simulink model "remoteMicrogrid"  (R2023a)
settings: Solver=FixedStepDiscrete  StartTime=0.0  StopTime=8  FixedStep=Ts  RelTol=1e-3
PreLoadFcn:
  | remoteMicrogridInputData
undefined symbols (not defined in the file): BESS, ControlRoom, DiscIntNeverNeededParam, Grid, Load, Machine, Microgrid, PV, T_on, Ts
libraries: ee_lib x46, eeGeneralControl x35, nesl_utility_internal x25, simulink x24, nesl_utility x20, fl_lib x17, slpidlib x12, eeTransforms x5, eeRmsMeasurement x4, eeTotalHarmonicDistorsion x4, eeSinusoidalMeasurement x3, batteryecm_lib x2
(part 5 of 5)

== system remoteMicrogrid/Operator Control Room/Measurements and visualizations /Resynchronization and Planned Islanding/Planned Islanding ==
  Grid Frequency : Inport
  Island Frequency : Inport  Port=2
  Grid Current : Inport  Port=3
  Island Voltage : Inport  Port=4
  Grid Voltage1 : Inport  Port=5
  PlannedIslandCommand : Inport  Port=6
  PlannedIsland : Inport  Port=7
  Power Tracking Command : Inport  Port=8
  BRK : Inport  Port=9
  " Grid and Island Voltage Frequency " : Scope  NumInputPorts=2
  Bus Creator1 : BusCreator  Inputs=2
  Bus Creator2 : BusCreator  Inputs=2
  Bus Creator3 : BusCreator  Inputs=4
  Bus Creator4 : BusCreator  Inputs=2
  "Grid Active & Reactive Power " : Subsystem
  Grid Voltage2 : InportShadow  Port=5
  Planned Islanding PCC voltage,Current : Scope  NumInputPorts=4
  wires:
  Bus Creator4/1 -> Planned Islanding PCC voltage,Current/4
  Bus Creator3/1 -> Planned Islanding PCC voltage,Current/1
  PlannedIslandCommand/1 -> Bus Creator3/1
  Grid Voltage2/1 -> Planned Islanding PCC voltage,Current/3, "Grid Active & Reactive Power "/1(Vabc)  "Grid Voltage"
  "Grid Active & Reactive Power "/2(Q) -> Bus Creator4/2  "Reactive Power (pu)"
  Grid Current/1 -> Planned Islanding PCC voltage,Current/2, "Grid Active & Reactive Power "/2(Iabc)
  "Grid Active & Reactive Power "/1(P) -> Bus Creator4/1  "Active Power (pu)"
  PlannedIsland/1 -> Bus Creator3/2
  Grid Frequency/1 -> Bus Creator1/1  "Grid Frequency"
  Island Frequency/1 -> Bus Creator1/2  "Island Frequency"
  Bus Creator1/1 -> " Grid and Island Voltage Frequency "/1
  Bus Creator2/1 -> " Grid and Island Voltage Frequency "/2
  Grid Voltage1/1 -> Bus Creator2/1  "Grid Voltage"
  Island Voltage/1 -> Bus Creator2/2  "Island Voltage"
  Power Tracking Command/1 -> Bus Creator3/3
  BRK/1 -> Bus Creator3/4

== system remoteMicrogrid/Operator Control Room/Measurements and visualizations /Resynchronization and Planned Islanding/Resync ==
  Grid Frequency : Inport
  Island Frequency : Inport  Port=2
  In1 : Inport  Port=3
  Grid Angle : Inport  Port=4
  Island Angle : Inport  Port=5
  Resynchronization : Inport  Port=6
  Grid Voltage : Inport  Port=7
  Grid Current : Inport  Port=8
  Island Voltage : Inport  Port=9
  Frequency Error : Inport  Port=10
  Grid Voltage1 : Inport  Port=11
  Phase Angle Error : Inport  Port=12
  Voltage Error : Inport  Port=13
  Bus Creator{,1..4} (5 alike) : BusCreator  Inputs=2
  "Grid Active & Reactive Power " : Subsystem
  Resynch and PCC voltage,Current : Scope  NumInputPorts=4
  Voltage and Frequency Matching : Scope  NumInputPorts=6
  wires:
  Grid Current/1 -> Resynch and PCC voltage,Current/2, "Grid Active & Reactive Power "/2(Iabc)
  Bus Creator1/1 -> Voltage and Frequency Matching/2
  Resynchronization/1 -> Bus Creator3/2
  Bus Creator3/1 -> Resynch and PCC voltage,Current/1
  "Grid Active & Reactive Power "/1(P) -> Bus Creator4/1  "Active Power (pu)"
  Island Voltage/1 -> Bus Creator2/2
  Grid Voltage1/1 -> Resynch and PCC voltage,Current/3, "Grid Active & Reactive Power "/1(Vabc)
  Bus Creator4/1 -> Resynch and PCC voltage,Current/4
  Bus Creator2/1 -> Voltage and Frequency Matching/3
  Bus Creator/1 -> Voltage and Frequency Matching/1
  Grid Frequency/1 -> Bus Creator/1
  Grid Angle/1 -> Bus Creator1/1
  Voltage Error/1 -> Voltage and Frequency Matching/6
  Island Frequency/1 -> Bus Creator/2
  Island Angle/1 -> Bus Creator1/2
  Phase Angle Error/1 -> Voltage and Frequency Matching/5
  Grid Voltage/1 -> Bus Creator2/1
  "Grid Active & Reactive Power "/2(Q) -> Bus Creator4/2  "Reactive Power (pu)"
  In1/1 -> Bus Creator3/1  "Resynch Command"
  Frequency Error/1 -> Voltage and Frequency Matching/4

== system remoteMicrogrid/Operator Control Room/Monitoring of system performance/Load /Subsystem4 ==
  Voltage : Inport
  Change Detector : eeGeneralControl/Change Detector  VariantControl=Variant1  LabelModeActiveChoice=Discrete  ChangeType=Rising edge  x0=0  Ts=Ts
  Change Detector1 : eeGeneralControl/Change Detector  VariantControl=Variant1  LabelModeActiveChoice=Discrete  ChangeType=Rising edge  x0=0  Ts=Ts
  Compare To Constant2 : simulink/Logic and Bit Operations/Compare To Constant  relop=<=  const=Microgrid.LoadVolatgeRMSLow  OutDataTypeStr=boolean
  Compare To Constant3 : simulink/Logic and Bit Operations/Compare To Constant  relop=>  const=Microgrid.LoadVolatgeRMSHigh  OutDataTypeStr=boolean
  VoltageLow : Outport
  VoltageHigh : Outport  Port=2
  wires:
  Change Detector/1 -> VoltageLow/1
  Compare To Constant2/1 -> Change Detector/1
  Voltage/1 -> Compare To Constant3/1, Compare To Constant2/1
  Change Detector1/1 -> VoltageHigh/1
  Compare To Constant3/1 -> Change Detector1/1

== system remoteMicrogrid/Operator Control Room/Monitoring of system performance/Load /start at 0.2 s2 ==
  In1 : Inport
  Constant : Constant  Value=0.707
  Step : Step  Time=0.3  SampleTime=Ts
  Switch : Switch  Criteria=u2 > Threshold  Threshold=0.5  SaturateOnIntegerOverflow=off  InputSameDT=off
  u : Outport
  wires:
  In1/1 -> Switch/1
  Switch/1 -> u/1
  Constant/1 -> Switch/3
  Step/1 -> Switch/2

== system remoteMicrogrid/Operator Control Room/Monitoring of system performance/Load /start at 0.2 s4 ==
  In1 : Inport
  Constant : Constant  Value=0.491
  Step : Step  Time=0.3  SampleTime=Ts
  Switch : Switch  Criteria=u2 > Threshold  Threshold=0.5  SaturateOnIntegerOverflow=off  InputSameDT=off
  u : Outport
  wires:
  In1/1 -> Switch/1
  Switch/1 -> u/1
  Constant/1 -> Switch/3
  Step/1 -> Switch/2

== system remoteMicrogrid/Operator Control Room/Monitoring of system performance/Load /start at 0.2 s5 ==
  In1 : Inport
  Constant : Constant  Value=75
  Step : Step  Time=0.3  SampleTime=Ts
  Switch : Switch  Criteria=u2 > Threshold  Threshold=0.5  SaturateOnIntegerOverflow=off  InputSameDT=off
  u : Outport
  wires:
  Step/1 -> Switch/2
  Constant/1 -> Switch/3
  Switch/1 -> u/1
  In1/1 -> Switch/1

== system remoteMicrogrid/Operator Control Room/Monitoring of system performance/Microgrid/Subsystem ==
  Frequency : Inport
  Change Detector : eeGeneralControl/Change Detector  VariantControl=Variant1  LabelModeActiveChoice=Discrete  ChangeType=Rising edge  x0=0  Ts=Ts
  Change Detector1 : eeGeneralControl/Change Detector  VariantControl=Variant1  LabelModeActiveChoice=Discrete  ChangeType=Rising edge  x0=0  Ts=Ts
  Compare To Constant2 : simulink/Logic and Bit Operations/Compare To Constant  relop=<  const=Microgrid.FrequencyLow  OutDataTypeStr=boolean
  Compare To Constant3 : simulink/Logic and Bit Operations/Compare To Constant  relop=>  const=Microgrid.FrequencyHigh  OutDataTypeStr=boolean
  FrequencyLow : Outport
  FrequencyHigh : Outport  Port=2
  wires:
  Change Detector/1 -> FrequencyLow/1
  Compare To Constant2/1 -> Change Detector/1
  Frequency/1 -> Compare To Constant3/1, Compare To Constant2/1
  Change Detector1/1 -> FrequencyHigh/1
  Compare To Constant3/1 -> Change Detector1/1

== system remoteMicrogrid/Operator Control Room/Monitoring of system performance/Microgrid/Subsystem3 ==
  Voltage : Inport
  Change Detector : eeGeneralControl/Change Detector  VariantControl=Variant1  LabelModeActiveChoice=Discrete  ChangeType=Rising edge  x0=0  Ts=Ts
  Change Detector1 : eeGeneralControl/Change Detector  VariantControl=Variant1  LabelModeActiveChoice=Discrete  ChangeType=Rising edge  x0=0  Ts=Ts
  Compare To Constant2 : simulink/Logic and Bit Operations/Compare To Constant  relop=<=  const=Microgrid.VoltageLow  OutDataTypeStr=boolean
  Compare To Constant3 : simulink/Logic and Bit Operations/Compare To Constant  relop=>  const=Microgrid.VoltageHigh  OutDataTypeStr=boolean
  VoltageLow : Outport
  VoltageHigh : Outport  Port=2
  wires:
  Compare To Constant3/1 -> Change Detector/1
  Change Detector/1 -> VoltageHigh/1
  Voltage/1 -> Compare To Constant2/1, Compare To Constant3/1
  Compare To Constant2/1 -> Change Detector1/1
  Change Detector1/1 -> VoltageLow/1

== system remoteMicrogrid/Operator Control Room/Monitoring of system performance/Microgrid/start at 2 s ==
  In1 : Inport
  Constant : Constant  Value=60
  Step : Step  Time=2  SampleTime=Ts
  Switch : Switch  Criteria=u2 > Threshold  Threshold=0.5  SaturateOnIntegerOverflow=off  InputSameDT=off
  u : Outport
  wires:
  Step/1 -> Switch/2
  Constant/1 -> Switch/3
  Switch/1 -> u/1
  In1/1 -> Switch/1

== system remoteMicrogrid/Operator Control Room/Monitoring of system performance/Microgrid/start at 2 s1 ==
  In1 : Inport
  Constant : Constant
  Step : Step  Time=2  SampleTime=Ts
  Switch : Switch  Criteria=u2 > Threshold  Threshold=0.5  SaturateOnIntegerOverflow=off  InputSameDT=off
  u : Outport
  wires:
  Step/1 -> Switch/2
  Constant/1 -> Switch/3
  Switch/1 -> u/1
  In1/1 -> Switch/1

== system remoteMicrogrid/Operator Control Room/Monitoring of system performance/Subsystem/start at 2.5 s ==
  ReactivePower : Inport
  Constant : Constant
  Step : Step  Time=2.5  SampleTime=Ts
  Switch : Switch  Criteria=u2 > Threshold  Threshold=0.5  SaturateOnIntegerOverflow=off  InputSameDT=off
  u : Outport
  wires:
  ReactivePower/1 -> Switch/1
  Switch/1 -> u/1
  Constant/1 -> Switch/3
  Step/1 -> Switch/2

== system remoteMicrogrid/Operator Control Room/Monitoring of system performance/Subsystem/start at 2.5 s1 ==
  ActivePower : Inport
  Constant : Constant
  Step : Step  Time=2.5  SampleTime=Ts
  Switch : Switch  Criteria=u2 > Threshold  Threshold=0.5  SaturateOnIntegerOverflow=off  InputSameDT=off
  u : Outport
  wires:
  Step/1 -> Switch/2
  Constant/1 -> Switch/3
  Switch/1 -> u/1
  ActivePower/1 -> Switch/1

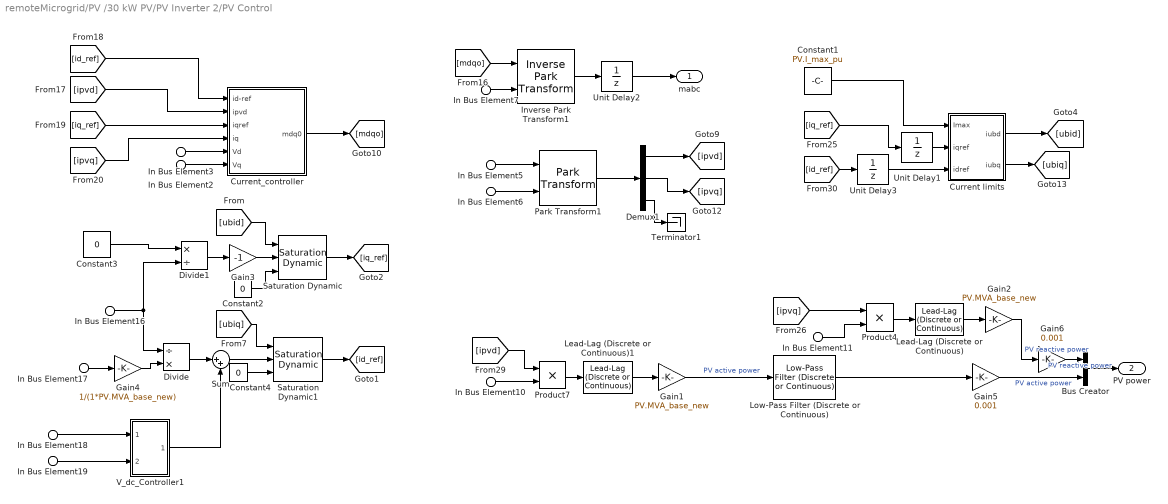
== system remoteMicrogrid/PV /30 kW PV/PV Inverter 2/PV Control ==
  In Bus Element17 : Inport  PortName=PV_plant1  Element=Pref1
  In Bus Element18 : Inport  PortName=PV_plant1  Element=Vdc_measured
  In Bus Element19 : Inport  PortName=PV_plant1  Element=Vdc_ref
  In Bus Element{3,10..11,16} (4 alike) : Inport  Port=2  PortName=PV  Element=Vd
  In Bus Element2 : Inport  Port=2  PortName=PV  Element=Vq
  In Bus Element6 : Inport  Port=2  PortName=PV  Element=Theta
  In Bus Element7 : Inport  Port=2  PortName=PV  Element=Theta
  In Bus Element5 : Inport  Port=3  PortName=ipv1  Element=1
  Bus Creator : BusCreator  Inputs=2
  Constant1 : Constant  Value=PV.I_max_pu
  Constant2 : Constant  Value=0
  Constant3 : Constant  Value=0
  Constant4 : Constant  Value=0
  Current limits : Subsystem
  Current_controller : Subsystem
  Demux1 : Demux  Outputs=3
  Divide : Product  Inputs=/*
  Divide1 : Product  Inputs=*/
  Gain1 : Gain  Gain=PV.MVA_base_new
  Gain2 : Gain  Gain=PV.MVA_base_new
  Gain3 : Gain  Gain=-1
  Gain4 : Gain  Gain=1/(1*PV.MVA_base_new)
  Gain5 : Gain  Gain=0.001
  Gain6 : Gain  Gain=0.001
  Inverse Park Transform1 : eeTransforms/Inverse Park Transform  AxisAlignment=Q-axis  PowerInvariant=off
  Lead-Lag (Discrete or Continuous) : eeGeneralControl/Lead-Lag (Discrete or Continuous)  T1=0  T2=PV.t_sensor  B=inf  A=-inf  init_option=Inherited from block input  x0=0  Ts=Ts
      settings: LibrarySourceBlock=|
      | ee_sl_lib/General Control/Lead-Lag
      | (Discrete or Continuous)
  Lead-Lag (Discrete or Continuous)1 : eeGeneralControl/Lead-Lag (Discrete or Continuous)  T1=0  T2=PV.t_sensor  B=inf  A=-inf  init_option=Inherited from block input  x0=0  Ts=Ts
      settings: LibrarySourceBlock=|
      | ee_sl_lib/General Control/Lead-Lag
      | (Discrete or Continuous)
  Low-Pass Filter (Discrete or Continuous) : eeGeneralControl/Low-Pass Filter (Discrete or Continuous)  K=1  T=0.02  B=inf  A=-inf  init_option=Inherited from block input  x0=0  Ts=-1
  Park Transform1 : eeTransforms/Park Transform  AxisAlignment=Q-axis  PowerInvariant=off
  Product4 : Product
  Product7 : Product
  Saturation Dynamic : simulink/Discontinuities/Saturation Dynamic  OutMin=[]  OutMax=[]  OutDataTypeStr=Inherit: Same as second input  OutDataType=fixdt(1, 16)  OutScaling=2^-10  DoSatur=off
  Saturation Dynamic1 : simulink/Discontinuities/Saturation Dynamic  OutMin=[]  OutMax=[]  OutDataTypeStr=Inherit: Same as second input  OutDataType=fixdt(1, 16)  OutScaling=2^-10  DoSatur=off
  Sum : Sum  Inputs=|++
  Terminator1 : Terminator
  Unit Delay1 : UnitDelay  SampleTime=Ts  HasFrameUpgradeWarning=on
  Unit Delay2 : UnitDelay  SampleTime=Ts  HasFrameUpgradeWarning=on
  Unit Delay3 : UnitDelay  SampleTime=Ts  HasFrameUpgradeWarning=on
  V_dc_Controller1 : Subsystem
  mabc : Outport
  PV power : Outport  Port=2
  wires:
  [id_ref] -> Unit Delay3/1
  Current limits/2(iubq) -> [ubiq]
  Gain1/1 -> Low-Pass Filter (Discrete or Continuous)/1  "PV active power"
  Product4/1 -> Lead-Lag (Discrete or Continuous)/1
  Product7/1 -> Lead-Lag (Discrete or Continuous)1/1
  In Bus Element2/1 -> Current_controller/6(Vq)
  Current_controller/1(mdq0) -> [mdqo]
  Constant1/1 -> Current limits/1(Imax)
  Inverse Park Transform1/1 -> Unit Delay2/1
  Demux1/2 -> [ipvq]
  Unit Delay2/1 -> mabc/1
  Demux1/1 -> [ipvd]
  [ipvq] -> Product4/1
  Demux1/3 -> Terminator1/1
  [mdqo] -> Inverse Park Transform1/1
  Current limits/1(iubd) -> [ubid]
  Park Transform1/1 -> Demux1/1
  [id_ref] -> Current_controller/1(id-ref)
  [iq_ref] -> Unit Delay1/1
  In Bus Element3/1 -> Current_controller/5(Vd)
  Unit Delay1/1 -> Current limits/2(iqref)
  [iq_ref] -> Current_controller/3(iqref)
  [ipvq] -> Current_controller/4(iq)
  In Bus Element10/1 -> Product7/2
  In Bus Element6/1 -> Park Transform1/2
  In Bus Element7/1 -> Inverse Park Transform1/2
  [ipvd] -> Product7/1
  Unit Delay3/1 -> Current limits/3(idref)
  In Bus Element11/1 -> Product4/2
  [ipvd] -> Current_controller/2(ipvd)
  Lead-Lag (Discrete or Continuous)1/1 -> Gain1/1
  Lead-Lag (Discrete or Continuous)/1 -> Gain2/1
  Gain2/1 -> Gain6/1  "PV reactive power"
  In Bus Element5/1 -> Park Transform1/1
  Constant4/1 -> Saturation Dynamic1/3
  V_dc_Controller1/1(Out1) -> Sum/2
  Constant2/1 -> Saturation Dynamic/3
  [ubiq] -> Saturation Dynamic1/1
  In Bus Element19/1 -> V_dc_Controller1/2(In2)
  Gain3/1 -> Saturation Dynamic/2
  In Bus Element18/1 -> V_dc_Controller1/1(PV_plant1)
  Gain4/1 -> Divide/2
  Sum/1 -> Saturation Dynamic1/2
  [ubid] -> Saturation Dynamic/1
  Constant3/1 -> Divide1/1
  In Bus Element16/1 -> Divide1/2, Divide/1
  Saturation Dynamic1/1 -> [id_ref]
  Divide/1 -> Sum/1
  Divide1/1 -> Gain3/1
  Saturation Dynamic/1 -> [iq_ref]
  In Bus Element17/1 -> Gain4/1
  Bus Creator/1 -> PV power/1
  Gain5/1 -> Bus Creator/2  "PV active power"
  Gain6/1 -> Bus Creator/1  "PV reactive power"
  Low-Pass Filter (Discrete or Continuous)/1 -> Gain5/1

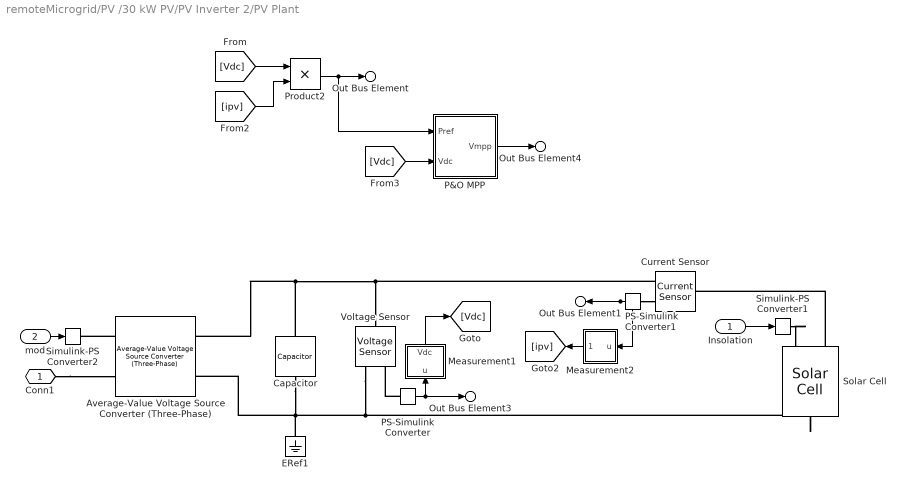
== system remoteMicrogrid/PV /30 kW PV/PV Inverter 2/PV Plant ==
  Insolation : Inport
  mod : Inport  Port=2
  Average-Value Voltage Source Converter (Three-Phase) : ee_lib/Semiconductors & Converters/Converters/Average-Value Voltage Source Converter (Three-Phase)  port_option=ee.enum.threePhasePort.composite  frequency_option=ee.enum.converters.frequency.variable  FRated=60 Hz  losses_parameterization=ee.enum.converters.losses.fixed  Pfixed=1 W  ks=0.01  kc1=1.7 V  kc2=0.01 Ohm  Ploss_vect=[100, 800, 1870, 3250, 4900] W  Irms_vect=[10, 100, 200, 300, 400] A  Vdc_nom=300 V  thermal_mass=30000 J/K  temperature_specify=off  temperature_priority=High  temperature=298.15 K  temperature_nominal_specify=off  temperature_nominal_unit=K  temperature_nominal_value=1
      settings: InternalSimscapePortConfiguration="{\"Bottom\":[],\"Left\":[{\"id\":\"ModWave\",\"label\":\"ModWave\",\"type\":\"input\"},{\"id\":\"N\",\"label\":\"~\",\"type\":\"foundation.electrical.three_phase\"}],\"Right\":[{\"id\":\"p\",\"label\":\"+\",\"type\":\"foundation.electrical.electrical\"},{\"id\":\"n\",\"label\":\"-\",\"type\":\"foundation.electrical.electrical\"}],\"Top\":[]}"
  Capacitor : fl_lib/Electrical/Electrical Elements/Capacitor  c=PV.C F  r=1e-6 Ohm  g=0 1/Ohm  i_specify=off  i_priority=None  i=0 A  i_nominal_specify=off  i_nominal_unit=A  i_nominal_value=1  v_specify=off  v_priority=None  v=6560*.5 V  v_nominal_specify=off  v_nominal_unit=V  v_nominal_value=1  vc_specify=on  vc_priority=None  vc=PV.Vdc V  vc_nominal_specify=off  vc_nominal_unit=V  vc_nominal_value=1
  Current Sensor : fl_lib/Electrical/Electrical Sensors/Current Sensor
  ERef1 : fl_lib/Electrical/Electrical Elements/Electrical Reference
  Measurement1 : Subsystem
  Measurement2 : Subsystem
  P&O MPP : Subsystem
  PS-Simulink Converter : nesl_utility/PS-Simulink Converter  PhysicalDomain=network_engine_domain  SubClassName=ps_output  LeftPortType=input  RightPortType=output  PseudoPeriodic=off  Frequencies=[]  VectorFormat=inherit  Unit=inherit  AffineConversion=off
  PS-Simulink Converter1 : nesl_utility/PS-Simulink Converter  PhysicalDomain=network_engine_domain  SubClassName=ps_output  LeftPortType=input  RightPortType=output  PseudoPeriodic=off  Frequencies=[]  VectorFormat=inherit  Unit=inherit  AffineConversion=off
  Product2 : Product
  Simulink-PS Converter1 : nesl_utility/Simulink-PS Converter  PhysicalDomain=network_engine_domain  SubClassName=ps_input  LeftPortType=input  RightPortType=output  PseudoPeriodic=off  Frequencies=[]  NoiseDistribution=none  NoiseParameters=[]  Unit=1  AffineConversion=off  FilteringAndDerivatives=provide  SimscapeFilterOrder=1  InputFilterTimeConstant=0.001  UdotUserProvided=0
  Simulink-PS Converter2 : nesl_utility/Simulink-PS Converter  PhysicalDomain=network_engine_domain  SubClassName=ps_input  LeftPortType=input  RightPortType=output  PseudoPeriodic=off  Frequencies=[]  NoiseDistribution=none  NoiseParameters=[]  Unit=1  AffineConversion=off  FilteringAndDerivatives=provide  SimscapeFilterOrder=1  InputFilterTimeConstant=0.001  UdotUserProvided=0
  Solar Cell : ee_lib/Sources/Solar Cell  prm=3  Isc=3.8 A  Voc=0.586 V  Is=Solar_cell.diode_saturation_current A  Is2=0 A  Iph=Solar_cell.solar_generated_current_AM A  Ir0=1000 W/m^2  ec=Solar_cell.quality_factor_i  N2=Solar_cell.quality_factor_j  Rs=Solar_cell.series_resistance Ohm  Rp=Solar_cell.parallel_resistance Ohm  N_series=PV.n_series_cell_panel*PV.n_series_panels_per_string  N_parallel=PV.n_parallel_strings_panel*PV.n_parallel_strings  TIPH1=Solar_cell.temp_cofficient 1/K  EG=Solar_cell.Eg eV  TXIS1=Solar_cell.temparature_exponent_Is1  TXIS2=Solar_cell.temparature_exponent_Is2  TRS1=Solar_cell.temparature_exponent_Rs  TRP1=Solar_cell.temparature_exponent_Rp  Tmeas=Solar_cell.measurement_temperature degC  TFIXED=Solar_cell.device_temperature degC  thermal_mass=100 J/K  initial_temperature=25 degC
  Voltage Sensor : fl_lib/Electrical/Electrical Sensors/Voltage Sensor
  Conn1 : PMIOPort  Side=Right
  Out Bus Element4 : Outport  PortName=PV_plant1  Element=Vdc_ref
  Out Bus Element : Outport  PortName=PV_plant1  Element=Pref1
  Out Bus Element3 : Outport  PortName=PV_plant1  Element=Vdc_measured
  Out Bus Element1 : Outport  PortName=PV_plant1  Element=ipv
  wires:
  PS-Simulink Converter1/1 -> Measurement2/1(u), Out Bus Element1/1
  Insolation/1 -> Simulink-PS Converter1/1
  [ipv] -> Product2/2
  PS-Simulink Converter/1 -> Measurement1/1(u), Out Bus Element3/1
  [Vdc] -> Product2/1
  mod/1 -> Simulink-PS Converter2/1
  Product2/1 -> P&O MPP/1(Pref), Out Bus Element/1
  P&O MPP/1(Vmpp) -> Out Bus Element4/1
  [Vdc] -> P&O MPP/2(Vdc)
  Measurement1/1(Vdc) -> [Vdc]
  Measurement2/1(Out1) -> [ipv]
  connections:
  PS-Simulink Converter/LConn1 -- Voltage Sensor/RConn1
  Capacitor/LConn1 -- Current Sensor/RConn2 -- Voltage Sensor/LConn1 -- Average-Value Voltage Source Converter (Three-Phase)/RConn1
  Voltage Sensor/RConn2 -- ERef1/LConn1 -- Capacitor/RConn1 -- Average-Value Voltage Source Converter (Three-Phase)/RConn2 -- Solar Cell/RConn1
  Average-Value Voltage Source Converter (Three-Phase)/LConn1 -- Simulink-PS Converter2/RConn1
  Solar Cell/LConn2 -- Current Sensor/LConn1
  Conn1/RConn1 -- Average-Value Voltage Source Converter (Three-Phase)/LConn2
  PS-Simulink Converter1/LConn1 -- Current Sensor/RConn1
  Simulink-PS Converter1/RConn1 -- Solar Cell/LConn1

== system remoteMicrogrid/Diesel Substation, BESS, & Microgrid Controller/Microgrid Controller/PLL/PLL/Subsystem ==
  In : Inport
  Bias : Bias  Bias=180  SaturateOnIntegerOverflow=off
  Bias1 : Bias  Bias=-180  SaturateOnIntegerOverflow=off
  Constant : Constant  Value=Grid.Frequency
  Constant1 : Constant  Value=360
  Data Type Conversion Inherited : simulink/Signal Attributes/Data Type Conversion Inherited  ConvertRealWorld=Real World Value  DoSatur=off
  Digital Clock : DigitalClock  SampleTime=Ts
  Mod : Math  Operator=mod
  Product : Product
  Sum : Sum  Inputs=+-  OutDataTypeStr=Inherit: Same as first input
  gain : Gain  Gain=2*pi
  rad2deg : Gain  Gain=180/pi
  Out : Outport
  wires:
  Data Type Conversion Inherited/1 -> Mod/2
  Sum/1 -> rad2deg/1
  rad2deg/1 -> Bias/1, Data Type Conversion Inherited/1
  Constant1/1 -> Data Type Conversion Inherited/2
  Digital Clock/1 -> Product/2
  Mod/1 -> Bias1/1
  Bias/1 -> Mod/1
  Constant/1 -> gain/1
  gain/1 -> Product/1
  In/1 -> Sum/1
  Product/1 -> Sum/2
  Bias1/1 -> Out/1

== system remoteMicrogrid/Diesel Substation, BESS, & Microgrid Controller/Microgrid Controller/PLL/PLL/start at 0.25 s ==
  In1 : Inport
  Constant : Constant  Value=60
  Step : Step  Time=0.25  SampleTime=Ts
  Switch : Switch  Criteria=u2 > Threshold  Threshold=0.5  SaturateOnIntegerOverflow=off  InputSameDT=off
  u : Outport
  wires:
  In1/1 -> Switch/1
  Switch/1 -> u/1
  Constant/1 -> Switch/3
  Step/1 -> Switch/2

== system remoteMicrogrid/Diesel Substation, BESS, & Microgrid Controller/Microgrid Controller/PLL/PLL/start at 0.25 s1 ==
  In1 : Inport
  Constant : Constant
  Step : Step  Time=0.25  SampleTime=Ts
  Switch : Switch  Criteria=u2 > Threshold  Threshold=0.5  SaturateOnIntegerOverflow=off  InputSameDT=off
  u : Outport
  wires:
  Step/1 -> Switch/2
  Constant/1 -> Switch/3
  Switch/1 -> u/1
  In1/1 -> Switch/1

== system remoteMicrogrid/Diesel Substation, BESS, & Microgrid Controller/Microgrid Controller/PLL/PLL1/Subsystem ==
  In : Inport
  Bias : Bias  Bias=180  SaturateOnIntegerOverflow=off
  Bias1 : Bias  Bias=-180  SaturateOnIntegerOverflow=off
  Constant : Constant  Value=Grid.Frequency
  Constant1 : Constant  Value=360
  Data Type Conversion Inherited : simulink/Signal Attributes/Data Type Conversion Inherited  ConvertRealWorld=Real World Value  DoSatur=off
  Digital Clock : DigitalClock  SampleTime=Ts
  Mod : Math  Operator=mod
  Product : Product
  Sum : Sum  Inputs=+-  OutDataTypeStr=Inherit: Same as first input
  gain : Gain  Gain=2*pi
  rad2deg : Gain  Gain=180/pi
  Out : Outport
  wires:
  Bias1/1 -> Out/1
  Product/1 -> Sum/2
  In/1 -> Sum/1
  gain/1 -> Product/1
  Constant/1 -> gain/1
  Bias/1 -> Mod/1
  Mod/1 -> Bias1/1
  Digital Clock/1 -> Product/2
  Constant1/1 -> Data Type Conversion Inherited/2
  rad2deg/1 -> Data Type Conversion Inherited/1, Bias/1
  Sum/1 -> rad2deg/1
  Data Type Conversion Inherited/1 -> Mod/2

== system remoteMicrogrid/Diesel Substation, BESS, & Microgrid Controller/Microgrid Controller/PLL/PLL1/start at 0.25 s ==
  In1 : Inport
  Constant : Constant
  Step : Step  Time=0.25  SampleTime=Ts
  Switch : Switch  Criteria=u2 > Threshold  Threshold=0.5  SaturateOnIntegerOverflow=off  InputSameDT=off
  u : Outport
  wires:
  Step/1 -> Switch/2
  Constant/1 -> Switch/3
  Switch/1 -> u/1
  In1/1 -> Switch/1

== system remoteMicrogrid/Diesel Substation, BESS, & Microgrid Controller/Microgrid Controller/PLL/PLL1/start at 0.25 s2 ==
  In1 : Inport
  Constant : Constant  Value=60
  Step : Step  Time=0.25  SampleTime=Ts
  Switch : Switch  Criteria=u2 > Threshold  Threshold=0.5  SaturateOnIntegerOverflow=off  InputSameDT=off
  u : Outport
  wires:
  In1/1 -> Switch/1
  Switch/1 -> u/1
  Constant/1 -> Switch/3
  Step/1 -> Switch/2

== system remoteMicrogrid/Diesel Substation, BESS, & Microgrid Controller/Microgrid Controller/Planned Island from Diesel/Control for Zero Powerflow for planned island/Planned Island Time Delay ==
  PlannedIsland : Inport
  PlannedislandCmd : Inport  Port=2
  Cast To Double : DataTypeConversion  OutDataTypeStr=double  SaturateOnIntegerOverflow=off  RndMeth=Floor
  Constant3 : Constant  Value=0
  Delay1 : Delay  DelayLength=500  SampleTime=Ts
  Delay2 : Delay  DelayLength=Microgrid.PlannedIslandDelay  InitialCondition=0  SampleTime=Ts*45
  Monostable Flip-Flop : eeGeneralControl/Monostable Flip-Flop  VariantControl=Variant1  LabelModeActiveChoice=Discrete  ChangeType=Rising edge  x0=0  Td=100  Ts=Ts
  Switch : Switch  Criteria=u2 > Threshold  Threshold=0.5  SaturateOnIntegerOverflow=off  InputSameDT=off
  MGController : Outport
  wires:
  PlannedislandCmd/1 -> Delay1/1
  PlannedIsland/1 -> Switch/1
  Monostable Flip-Flop/1 -> Cast To Double/1
  Delay2/1 -> MGController/1
  Delay1/1 -> Switch/2
  Constant3/1 -> Switch/3
  Cast To Double/1 -> Delay2/1
  Switch/1 -> Monostable Flip-Flop/1

== system remoteMicrogrid/Diesel Substation, BESS, & Microgrid Controller/Microgrid Controller/Resynchronization to Diesel/Frequency and voltage matching/Resynchronization Time Delay ==
  Resynchronization : Inport
  ResynchronizationCmd : Inport  Port=2
  Cast To Double : DataTypeConversion  OutDataTypeStr=double  SaturateOnIntegerOverflow=off  RndMeth=Floor
  Constant3 : Constant  Value=0
  Delay1 : Delay  DelayLength=500  SampleTime=Ts
  Delay2 : Delay  DelayLength=Microgrid.ResynchDelay  InitialCondition=0  SampleTime=Ts*45
  Monostable Flip-Flop : eeGeneralControl/Monostable Flip-Flop  VariantControl=Variant1  LabelModeActiveChoice=Discrete  ChangeType=Rising edge  x0=0  Td=100  Ts=Ts
      settings: LibrarySourceBlock=ee_sl_lib/General Control/Monostable Flip-Flop
  Switch : Switch  Criteria=u2 > Threshold  Threshold=0.5  SaturateOnIntegerOverflow=off  InputSameDT=off
  MGController : Outport
  wires:
  Switch/1 -> Monostable Flip-Flop/1
  Cast To Double/1 -> Delay2/1
  Constant3/1 -> Switch/3
  Delay1/1 -> Switch/2
  Delay2/1 -> MGController/1
  Monostable Flip-Flop/1 -> Cast To Double/1
  Resynchronization/1 -> Switch/1
  ResynchronizationCmd/1 -> Delay1/1

== system remoteMicrogrid/Diesel Substation, BESS, & Microgrid Controller/Microgrid Controller/Resynchronization to Diesel/Frequency and voltage matching/Synch Voltage ==
  MicrogridController : Inport
  ControlRoom : Inport  Port=2
  ReactivePower : Inport  Port=3
  Resynch : Inport  Port=4
  Gain1 : Gain  Gain=Microgrid.Kdroop
  Logical Operator1 : Logic  Operator=NOT  AllPortsSameDT=off  OutDataTypeStr=boolean
  Low-Pass Filter (Discrete or Continuous) : eeGeneralControl/Low-Pass Filter (Discrete or Continuous)  K=1  T=0.08  B=inf  A=-inf  init_option=Specify as parameter  x0=0  Ts=5*Ts
  Signal Sample and Hold : eeGeneralControl/Signal Sample and Hold  LabelModeActiveChoice=Discrete  x0=0  Ts=Ts
      settings: LibrarySourceBlock=ee_sl_lib/General Control/Signal Sample and Hold
  Subsystem2 : Subsystem
  Sum4 : Sum  Inputs=+-
  SynchVoltage : Outport
  wires:
  Low-Pass Filter (Discrete or Continuous)/1 -> Gain1/1
  Resynch/1 -> Logical Operator1/1
  Signal Sample and Hold/1 -> Sum4/1
  Gain1/1 -> Sum4/2
  Logical Operator1/1 -> Signal Sample and Hold/2
  MicrogridController/1 -> Subsystem2/1(MicrogridController)
  Subsystem2/1(SynchVoltage) -> Signal Sample and Hold/1
  Sum4/1 -> SynchVoltage/1
  ControlRoom/1 -> Subsystem2/2(ControlRoom)
  ReactivePower/1 -> Low-Pass Filter (Discrete or Continuous)/1

== system remoteMicrogrid/Operator Control Room/Measurements and visualizations /BESS, PV and Load Measurements/BESS and PV Measurements/Inverter Active & Reactive Power  ==
  Vabc : Inport
  Iabc : Inport  Port=2
  Demux : Demux  Outputs=3
  Gain : Gain  Gain=1/sqrt(3)
  Low-Pass Filter (Discrete or Continuous) : eeGeneralControl/Low-Pass Filter (Discrete or Continuous)  K=1  T=0.02  B=inf  A=-inf  init_option=Inherited from block input  x0=0  Ts=-1
  Low-Pass Filter (Discrete or Continuous)1 : eeGeneralControl/Low-Pass Filter (Discrete or Continuous)  K=1  T=0.02  B=inf  A=-inf  init_option=Inherited from block input  x0=0  Ts=-1
  Minus : Sum  Inputs=+-
  Minus1 : Sum  Inputs=+-
  Minus2 : Sum  Inputs=+-
  Mux : Mux  Inputs=3
  Product : Product
  Product1 : Product
  Sum of Elements : Sum  Inputs=+
  Sum of Elements1 : Sum  Inputs=+
  gain : Gain  Gain=2/3
  gain1 : Gain  Gain=2/3
  P : Outport  VectorParamsAs1DForOutWhenUnconnected=off
  Q : Outport  Port=2  VectorParamsAs1DForOutWhenUnconnected=off
  wires:
  Minus/1 -> Mux/3
  Minus2/1 -> Mux/2
  Minus1/1 -> Mux/1
  Gain/1 -> Low-Pass Filter (Discrete or Continuous)1/1
  Sum of Elements1/1 -> Gain/1
  Product1/1 -> Sum of Elements1/1
  Mux/1 -> Product1/2
  Demux/3 -> Minus1/2, Minus2/1
  Demux/2 -> Minus/2, Minus1/1
  Demux/1 -> Minus/1, Minus2/2
  Sum of Elements/1 -> Low-Pass Filter (Discrete or Continuous)/1
  Product/1 -> Sum of Elements/1
  Iabc/1 -> Product/2, Product1/1
  Vabc/1 -> Product/1, Demux/1
  Low-Pass Filter (Discrete or Continuous)/1 -> gain/1
  Low-Pass Filter (Discrete or Continuous)1/1 -> gain1/1
  gain/1 -> P/1  "BESS Active Power(pu)"
  gain1/1 -> Q/1  "BESS Reactive Power(pu)"

== system remoteMicrogrid/Operator Control Room/Measurements and visualizations /Resynchronization and Planned Islanding/Planned Islanding/Grid Active & Reactive Power  ==
  Vabc : Inport
  Iabc : Inport  Port=2
  Demux : Demux  Outputs=3
  Gain : Gain  Gain=1/sqrt(3)
  Low-Pass Filter (Discrete or Continuous) : eeGeneralControl/Low-Pass Filter (Discrete or Continuous)  K=1  T=0.02  B=inf  A=-inf  init_option=Inherited from block input  x0=0  Ts=-1
  Low-Pass Filter (Discrete or Continuous)1 : eeGeneralControl/Low-Pass Filter (Discrete or Continuous)  K=1  T=0.02  B=inf  A=-inf  init_option=Inherited from block input  x0=0  Ts=-1
  Minus : Sum  Inputs=+-
  Minus1 : Sum  Inputs=+-
  Minus2 : Sum  Inputs=+-
  Mux : Mux  Inputs=3
  Product : Product
  Product1 : Product
  Sum of Elements : Sum  Inputs=+
  Sum of Elements1 : Sum  Inputs=+
  gain : Gain  Gain=2/3
  gain1 : Gain  Gain=2/3
  P : Outport  VectorParamsAs1DForOutWhenUnconnected=off
  Q : Outport  Port=2  VectorParamsAs1DForOutWhenUnconnected=off
  wires:
  Minus/1 -> Mux/3
  Minus2/1 -> Mux/2
  Minus1/1 -> Mux/1
  Gain/1 -> Low-Pass Filter (Discrete or Continuous)1/1
  Sum of Elements1/1 -> Gain/1
  Product1/1 -> Sum of Elements1/1
  Mux/1 -> Product1/2
  Demux/3 -> Minus1/2, Minus2/1
  Demux/2 -> Minus/2, Minus1/1
  Demux/1 -> Minus/1, Minus2/2
  Sum of Elements/1 -> Low-Pass Filter (Discrete or Continuous)/1
  Product/1 -> Sum of Elements/1
  Iabc/1 -> Product/2, Product1/1
  Vabc/1 -> Product/1, Demux/1
  Low-Pass Filter (Discrete or Continuous)/1 -> gain/1
  Low-Pass Filter (Discrete or Continuous)1/1 -> gain1/1
  gain/1 -> P/1  "BESS Active Power(pu)"
  gain1/1 -> Q/1  "BESS Reactive Power(pu)"

== system remoteMicrogrid/Operator Control Room/Measurements and visualizations /Resynchronization and Planned Islanding/Resync/Grid Active & Reactive Power  ==
  Vabc : Inport
  Iabc : Inport  Port=2
  Demux : Demux  Outputs=3
  Gain : Gain  Gain=1/sqrt(3)
  Low-Pass Filter (Discrete or Continuous) : eeGeneralControl/Low-Pass Filter (Discrete or Continuous)  K=1  T=0.02  B=inf  A=-inf  init_option=Inherited from block input  x0=0  Ts=-1
  Low-Pass Filter (Discrete or Continuous)1 : eeGeneralControl/Low-Pass Filter (Discrete or Continuous)  K=1  T=0.02  B=inf  A=-inf  init_option=Inherited from block input  x0=0  Ts=-1
  Minus : Sum  Inputs=+-
  Minus1 : Sum  Inputs=+-
  Minus2 : Sum  Inputs=+-
  Mux : Mux  Inputs=3
  Product : Product
  Product1 : Product
  Sum of Elements : Sum  Inputs=+
  Sum of Elements1 : Sum  Inputs=+
  gain : Gain  Gain=2/3
  gain1 : Gain  Gain=2/3
  P : Outport  VectorParamsAs1DForOutWhenUnconnected=off
  Q : Outport  Port=2  VectorParamsAs1DForOutWhenUnconnected=off
  wires:
  Minus/1 -> Mux/3
  Minus2/1 -> Mux/2
  Minus1/1 -> Mux/1
  Gain/1 -> Low-Pass Filter (Discrete or Continuous)1/1
  Sum of Elements1/1 -> Gain/1
  Product1/1 -> Sum of Elements1/1
  Mux/1 -> Product1/2
  Demux/3 -> Minus1/2, Minus2/1
  Demux/2 -> Minus/2, Minus1/1
  Demux/1 -> Minus/1, Minus2/2
  Sum of Elements/1 -> Low-Pass Filter (Discrete or Continuous)/1
  Product/1 -> Sum of Elements/1
  Iabc/1 -> Product/2, Product1/1
  Vabc/1 -> Product/1, Demux/1
  Low-Pass Filter (Discrete or Continuous)/1 -> gain/1
  Low-Pass Filter (Discrete or Continuous)1/1 -> gain1/1
  gain/1 -> P/1  "BESS Active Power(pu)"
  gain1/1 -> Q/1  "BESS Reactive Power(pu)"

== system remoteMicrogrid/PV /30 kW PV/PV Inverter 2/PV Control/Current limits ==
  Imax : Inport
  iqref : Inport  Port=2
  idref : Inport  Port=3
  Constant8 : Constant  Value=0
  Constant9 : Constant  Value=0
  Sqrt : Sqrt
  Sqrt1 : Sqrt
  Square{1..4} (4 alike) : Math  Operator=square
  Step2 : Step  Time=T_on  SampleTime=Ts
  Step3 : Step  Time=T_on  SampleTime=Ts
  Sum6 : Sum  Inputs=|+-
  Sum9 : Sum  Inputs=|+-
  Switch1 : Switch  Threshold=.01  SaturateOnIntegerOverflow=off  InputSameDT=off
  Switch2 : Switch  Threshold=.01  SaturateOnIntegerOverflow=off  InputSameDT=off
  iubd : Outport
  iubq : Outport  Port=2
  wires:
  Sum9/1 -> Switch2/1
  Step3/1 -> Switch2/2
  Step2/1 -> Switch1/2
  Switch2/1 -> Sqrt1/1
  Square1/1 -> Sum6/1
  Switch1/1 -> Sqrt/1
  iqref/1 -> Square2/1
  Square3/1 -> Sum9/1
  Sum6/1 -> Switch1/1
  Square2/1 -> Sum6/2
  Constant8/1 -> Switch1/3
  Square4/1 -> Sum9/2
  Constant9/1 -> Switch2/3
  Sqrt/1 -> iubd/1
  Imax/1 -> Square3/1, Square1/1
  Sqrt1/1 -> iubq/1
  idref/1 -> Square4/1

== system remoteMicrogrid/PV /30 kW PV/PV Inverter 2/PV Control/Current_controller ==
  id-ref : Inport
  ipvd : Inport  Port=2
  iqref : Inport  Port=3
  iq : Inport  Port=4
  Vd : Inport  Port=5
  Vq : Inport  Port=6
  Constant4 : Constant  Value=0
  Gain1 : Gain  Gain=2*1*pi*60*PV.L/PV.z_base
  Gain2 : Gain  Gain=2*1*pi*60*PV.L/PV.z_base
  Mux1 : Mux  Inputs=3
  PID Controller : slpidlib/PID Controller  Controller=PID  Form=Parallel  TimeDomain=Discrete-time  UseExternalTs=off  SampleTime=-1  IntegratorMethod=Forward Euler  FilterMethod=Forward Euler  ControllerParametersSource=internal  P=PV.Kp_ic  I=PV.Ki_ic  UseKiTs=off  D=PV.Kd  N=100  UseFilter=on  TunerSelectOption=Transfer Function Based (PID Tuner App)  InitialConditionSource=internal  InitialConditionForIntegrator=0.9  InitialConditionForFilter=0  DifferentiatorICPrevScaledInput=0  ExternalReset=none  TrackingMode=off  Kt=1  LimitOutput=off  SatLimitsSource=internal  UpperSaturationLimit=inf  LowerSaturationLimit=-inf  LinearizeAsGain=on  AntiWindupMode=none  Kb=1  LimitIntegrator=off  UpperIntegratorSaturationLimit=inf  LowerIntegratorSaturationLimit=-inf  POutMin=[]  POutMax=[]  IOutMin=[]  IOutMax=[]  DOutMin=[]  DOutMax=[]  NOutMin=[]  NOutMax=[]  SumOutMin=[]  SumOutMax=[]  SaturationOutMin=[]  SaturationOutMax=[]  PParamMin=[]  PParamMax=[]  IParamMin=[]  IParamMax=[]  DParamMin=[]  DParamMax=[]  NParamMin=[]  NParamMax=[]  KbParamMin=[]  KbParamMax=[]  KtParamMin=[]  KtParamMax=[]  KbOutMin=[]  KbOutMax=[]  KtOutMin=[]  KtOutMax=[]  IntegratorOutMin=[]  IntegratorOutMax=[]  FilterOutMin=[]  FilterOutMax=[]  SumI1OutMin=[]  SumI1OutMax=[]  SumI2OutMin=[]  SumI2OutMax=[]  SumI3OutMin=[]  SumI3OutMax=[]  SumI4OutMin=[]  SumI4OutMax=[]  SumDOutMin=[]  SumDOutMax=[]  DifferentiatorOutMin=[]  DifferentiatorOutMax=[]  FilterDiffOutCoefMin=[]  FilterDiffOutCoefMax=[]  ReciprocalOutMin=[]  ReciprocalOutMax=[]  SumDenOutMin=[]  SumDenOutMax=[]  SumNumOutMin=[]  SumNumOutMax=[]  DivideOutMin=[]  DivideOutMax=[]  UdiffTsProdOutMin=[]  UdiffTsProdOutMax=[]  NTsProdOutMin=[]  NTsProdOutMax=[]  UintegralTsProdOutMin=[]  UintegralTsProdOutMax=[]  UngainTsProdOutMin=[]  UngainTsProdOutMax=[]  ClampingZeroOutDataTypeStr=Inherit: Inherit via back propagation  ClampingZeroOutMin=[]  ClampingZeroOutMax=[]  FilterDenConstantOutDataTypeStr=Inherit: Inherit via back propagation  FilterDenConstantOutMin=[]  FilterDenConstantOutMax=[]  PCopyOutDataTypeStr=Inherit: Inherit via back propagation  PCopyOutMin=[]  PCopyOutMax=[]  NCopyOutDataTypeStr=Inherit: Inherit via back propagation  NCopyOutMin=[]  NCopyOutMax=[]  IntegratorContinuousStateAttributes=''  IntegratorStateMustResolveToSignalObject=off  IntegratorRTWStateStorageClass=Auto  FilterContinuousStateAttributes=''  FilterStateMustResolveToSignalObject=off  FilterRTWStateStorageClass=Auto  ParallelPVariant=InternalParameters  IdealPVariant=Disabled  IVariant=InternalParameters  DVariant=InternalParameters  IntegratorVariant=Discrete  SatVariant=Disabled  AWVariant=Passthrough  PCopyVariant=Disabled  TRVariant=Disabled  FdbkBlocksVariant=Forward  IdealPFdbkVariant=Disabled  SatFdbkVariant=Disabled  DerivativeFilterVariant=ForwardEulerFilter  NVariant=InternalParameters  NCopyVariant=Disabled  FilterICVariant=InternalICsFilter  IntegratorICVariant=InternalICs  ExternalResetVariant=Disabled  TRSumVariant=Passthrough  SumFdbkVariant=Disabled  SumVariant=Sum_PID  TsampFilterVariant=InternalTs  TsampNgainVariant=Passthrough  TsampIntegralVariant=Disabled_SignalSpec  ExternalSaturationOutDataTypeStr=Inherit: Same as second input
  PID Controller1 : slpidlib/PID Controller  Controller=PID  Form=Parallel  TimeDomain=Discrete-time  UseExternalTs=off  SampleTime=-1  IntegratorMethod=Forward Euler  FilterMethod=Forward Euler  ControllerParametersSource=internal  P=PV.Kp_ic  I=PV.Ki_ic  UseKiTs=off  D=PV.Kd  N=100  UseFilter=on  TunerSelectOption=Transfer Function Based (PID Tuner App)  InitialConditionSource=internal  InitialConditionForIntegrator=1.05  InitialConditionForFilter=0  DifferentiatorICPrevScaledInput=0  ExternalReset=none  TrackingMode=off  Kt=1  LimitOutput=off  SatLimitsSource=internal  UpperSaturationLimit=inf  LowerSaturationLimit=-inf  LinearizeAsGain=on  AntiWindupMode=none  Kb=1  LimitIntegrator=off  UpperIntegratorSaturationLimit=inf  LowerIntegratorSaturationLimit=-inf  POutMin=[]  POutMax=[]  IOutMin=[]  IOutMax=[]  DOutMin=[]  DOutMax=[]  NOutMin=[]  NOutMax=[]  SumOutMin=[]  SumOutMax=[]  SaturationOutMin=[]  SaturationOutMax=[]  PParamMin=[]  PParamMax=[]  IParamMin=[]  IParamMax=[]  DParamMin=[]  DParamMax=[]  NParamMin=[]  NParamMax=[]  KbParamMin=[]  KbParamMax=[]  KtParamMin=[]  KtParamMax=[]  KbOutMin=[]  KbOutMax=[]  KtOutMin=[]  KtOutMax=[]  IntegratorOutMin=[]  IntegratorOutMax=[]  FilterOutMin=[]  FilterOutMax=[]  SumI1OutMin=[]  SumI1OutMax=[]  SumI2OutMin=[]  SumI2OutMax=[]  SumI3OutMin=[]  SumI3OutMax=[]  SumI4OutMin=[]  SumI4OutMax=[]  SumDOutMin=[]  SumDOutMax=[]  DifferentiatorOutMin=[]  DifferentiatorOutMax=[]  FilterDiffOutCoefMin=[]  FilterDiffOutCoefMax=[]  ReciprocalOutMin=[]  ReciprocalOutMax=[]  SumDenOutMin=[]  SumDenOutMax=[]  SumNumOutMin=[]  SumNumOutMax=[]  DivideOutMin=[]  DivideOutMax=[]  UdiffTsProdOutMin=[]  UdiffTsProdOutMax=[]  NTsProdOutMin=[]  NTsProdOutMax=[]  UintegralTsProdOutMin=[]  UintegralTsProdOutMax=[]  UngainTsProdOutMin=[]  UngainTsProdOutMax=[]  ClampingZeroOutDataTypeStr=Inherit: Inherit via back propagation  ClampingZeroOutMin=[]  ClampingZeroOutMax=[]  FilterDenConstantOutDataTypeStr=Inherit: Inherit via back propagation  FilterDenConstantOutMin=[]  FilterDenConstantOutMax=[]  PCopyOutDataTypeStr=Inherit: Inherit via back propagation  PCopyOutMin=[]  PCopyOutMax=[]  NCopyOutDataTypeStr=Inherit: Inherit via back propagation  NCopyOutMin=[]  NCopyOutMax=[]  IntegratorContinuousStateAttributes=''  IntegratorStateMustResolveToSignalObject=off  IntegratorRTWStateStorageClass=Auto  FilterContinuousStateAttributes=''  FilterStateMustResolveToSignalObject=off  FilterRTWStateStorageClass=Auto  ParallelPVariant=InternalParameters  IdealPVariant=Disabled  IVariant=InternalParameters  DVariant=InternalParameters  IntegratorVariant=Discrete  SatVariant=Disabled  AWVariant=Passthrough  PCopyVariant=Disabled  TRVariant=Disabled  FdbkBlocksVariant=Forward  IdealPFdbkVariant=Disabled  SatFdbkVariant=Disabled  DerivativeFilterVariant=ForwardEulerFilter  NVariant=InternalParameters  NCopyVariant=Disabled  FilterICVariant=InternalICsFilter  IntegratorICVariant=InternalICs  ExternalResetVariant=Disabled  TRSumVariant=Passthrough  SumFdbkVariant=Disabled  SumVariant=Sum_PID  TsampFilterVariant=InternalTs  TsampNgainVariant=Passthrough  TsampIntegralVariant=Disabled_SignalSpec  ExternalSaturationOutDataTypeStr=Inherit: Same as second input
  Sum1 : Sum  Inputs=|+-
  Sum3 : Sum  Inputs=|++-
  Sum4 : Sum  Inputs=|+++
  Sum5 : Sum  Inputs=|+-
  mdq0 : Outport
  wires:
  PID Controller/1 -> Sum3/2
  Sum3/1 -> Mux1/1
  Gain2/1 -> Sum3/3
  ipvd/1 -> Gain1/1, Sum1/2
  id-ref/1 -> Sum1/1
  Gain1/1 -> Sum4/3
  Vq/1 -> Sum4/2
  iq/1 -> Gain2/1, Sum5/2
  Sum1/1 -> PID Controller/1
  Vd/1 -> Sum3/1
  Constant4/1 -> Mux1/3
  Sum5/1 -> PID Controller1/1
  iqref/1 -> Sum5/1
  PID Controller1/1 -> Sum4/1
  Sum4/1 -> Mux1/2
  Mux1/1 -> mdq0/1

== system remoteMicrogrid/PV /30 kW PV/PV Inverter 2/PV Control/V_dc_Controller1 ==
  PV_plant1 : Inport
  In2 : Inport  Port=2
  Gain : Gain  Gain=1/PV.Vdc_base
  PID Controller : slpidlib/PID Controller  Controller=PID  Form=Parallel  TimeDomain=Discrete-time  UseExternalTs=off  SampleTime=-1  IntegratorMethod=Forward Euler  FilterMethod=Forward Euler  ControllerParametersSource=internal  P=PV.Kp_v  I=PV.Ki_v  UseKiTs=off  D=PV.Kd_v  N=100  UseFilter=on  TunerSelectOption=Transfer Function Based (PID Tuner App)  ZeroCross=off  InitialConditionSource=internal  InitialConditionForIntegrator=0  InitialConditionForFilter=0  DifferentiatorICPrevScaledInput=0  ExternalReset=none  TrackingMode=off  Kt=1  LimitOutput=off  SatLimitsSource=internal  UpperSaturationLimit=inf  LowerSaturationLimit=-inf  LinearizeAsGain=on  AntiWindupMode=none  Kb=1  LimitIntegrator=off  UpperIntegratorSaturationLimit=inf  LowerIntegratorSaturationLimit=-inf  POutMin=[]  POutMax=[]  IOutMin=[]  IOutMax=[]  DOutMin=[]  DOutMax=[]  NOutMin=[]  NOutMax=[]  SumOutMin=[]  SumOutMax=[]  SaturationOutMin=[]  SaturationOutMax=[]  PParamMin=[]  PParamMax=[]  IParamMin=[]  IParamMax=[]  DParamMin=[]  DParamMax=[]  NParamMin=[]  NParamMax=[]  KbParamMin=[]  KbParamMax=[]  KtParamMin=[]  KtParamMax=[]  KbOutMin=[]  KbOutMax=[]  KtOutMin=[]  KtOutMax=[]  IntegratorOutMin=[]  IntegratorOutMax=[]  FilterOutMin=[]  FilterOutMax=[]  SumI1OutMin=[]  SumI1OutMax=[]  SumI2OutMin=[]  SumI2OutMax=[]  SumI3OutMin=[]  SumI3OutMax=[]  SumI4OutMin=[]  SumI4OutMax=[]  SumDOutMin=[]  SumDOutMax=[]  DifferentiatorOutMin=[]  DifferentiatorOutMax=[]  FilterDiffOutCoefMin=[]  FilterDiffOutCoefMax=[]  ReciprocalOutMin=[]  ReciprocalOutMax=[]  SumDenOutMin=[]  SumDenOutMax=[]  SumNumOutMin=[]  SumNumOutMax=[]  DivideOutMin=[]  DivideOutMax=[]  UdiffTsProdOutMin=[]  UdiffTsProdOutMax=[]  NTsProdOutMin=[]  NTsProdOutMax=[]  UintegralTsProdOutMin=[]  UintegralTsProdOutMax=[]  UngainTsProdOutMin=[]  UngainTsProdOutMax=[]  ClampingZeroOutDataTypeStr=Inherit: Inherit via back propagation  ClampingZeroOutMin=[]  ClampingZeroOutMax=[]  FilterDenConstantOutDataTypeStr=Inherit: Inherit via back propagation  FilterDenConstantOutMin=[]  FilterDenConstantOutMax=[]  PCopyOutDataTypeStr=Inherit: Inherit via back propagation  PCopyOutMin=[]  PCopyOutMax=[]  NCopyOutDataTypeStr=Inherit: Inherit via back propagation  NCopyOutMin=[]  NCopyOutMax=[]  IntegratorContinuousStateAttributes=''  IntegratorStateMustResolveToSignalObject=off  IntegratorRTWStateStorageClass=Auto  FilterContinuousStateAttributes=''  FilterStateMustResolveToSignalObject=off  FilterRTWStateStorageClass=Auto  ParallelPVariant=InternalParameters  IdealPVariant=Disabled  IVariant=InternalParameters  DVariant=InternalParameters  IntegratorVariant=Discrete  SatVariant=Disabled  AWVariant=Passthrough  PCopyVariant=Disabled  TRVariant=Disabled  FdbkBlocksVariant=Forward  IdealPFdbkVariant=Disabled  SatFdbkVariant=Disabled  DerivativeFilterVariant=ForwardEulerFilter  NVariant=InternalParameters  NCopyVariant=Disabled  FilterICVariant=InternalICsFilter  IntegratorICVariant=InternalICs  ExternalResetVariant=Disabled  TRSumVariant=Passthrough  SumFdbkVariant=Disabled  SumVariant=Sum_PID  TsampFilterVariant=InternalTs  TsampNgainVariant=Passthrough  TsampIntegralVariant=Disabled_SignalSpec  ExternalSaturationOutDataTypeStr=Inherit: Same as second input
  Sum : Sum  Inputs=|+-
  Out1 : Outport
  wires:
  PV_plant1/1 -> Sum/1
  In2/1 -> Sum/2
  PID Controller/1 -> Out1/1
  Gain/1 -> PID Controller/1
  Sum/1 -> Gain/1

== system remoteMicrogrid/PV /30 kW PV/PV Inverter 2/PV Plant/Measurement1 ==
  u : Inport
  Lead-Lag (Discrete or Continuous) : eeGeneralControl/Lead-Lag (Discrete or Continuous)  T1=0  T2=PV.t_sensor  B=inf  A=-inf  init_option=Inherited from block input  x0=0  Ts=Ts
      settings: LibrarySourceBlock=|
      | ee_sl_lib/General Control/Lead-Lag
      | (Discrete or Continuous)
  Vdc : Outport
  wires:
  Lead-Lag (Discrete or Continuous)/1 -> Vdc/1
  u/1 -> Lead-Lag (Discrete or Continuous)/1

== system remoteMicrogrid/PV /30 kW PV/PV Inverter 2/PV Plant/Measurement2 ==
  u : Inport
  Lead-Lag (Discrete or Continuous) : eeGeneralControl/Lead-Lag (Discrete or Continuous)  T1=0  T2=PV.t_sensor  B=inf  A=-inf  init_option=Inherited from block input  x0=0  Ts=Ts
      settings: LibrarySourceBlock=|
      | ee_sl_lib/General Control/Lead-Lag
      | (Discrete or Continuous)
  Out1 : Outport
  wires:
  Lead-Lag (Discrete or Continuous)/1 -> Out1/1
  u/1 -> Lead-Lag (Discrete or Continuous)/1

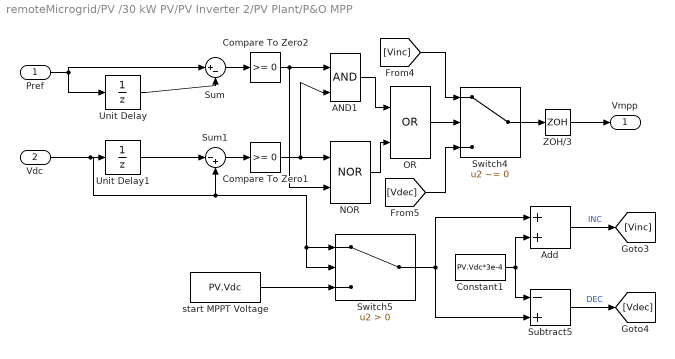
== system remoteMicrogrid/PV /30 kW PV/PV Inverter 2/PV Plant/P&O MPP ==
  Pref : Inport
  Vdc : Inport  Port=2
  AND1 : Logic  IconShape=distinctive  AllPortsSameDT=off  OutDataTypeStr=boolean
  Add : Sum
  Compare To Zero1 : simulink/Logic and Bit Operations/Compare To Zero  relop=>=  OutDataTypeStr=boolean
  Compare To Zero2 : simulink/Logic and Bit Operations/Compare To Zero  relop=>=  OutDataTypeStr=boolean
  Constant1 : Constant  Value=PV.Vdc*3e-4
  NOR : Logic  Operator=NOR  IconShape=distinctive  AllPortsSameDT=off  OutDataTypeStr=boolean
  OR : Logic  Operator=OR  IconShape=distinctive  AllPortsSameDT=off  OutDataTypeStr=boolean
  Subtract5 : Sum  Inputs=-+
  Sum : Sum  Inputs=|+-
  Sum1 : Sum  Inputs=|-+
  Switch4 : Switch  Criteria=u2 ~= 0  SaturateOnIntegerOverflow=off  InputSameDT=off
  Switch5 : Switch  Criteria=u2 > Threshold  SaturateOnIntegerOverflow=off  InputSameDT=off
  Unit Delay : UnitDelay  InitialCondition=PV.Vdc  SampleTime=10*Ts  HasFrameUpgradeWarning=on
  Unit Delay1 : UnitDelay  InitialCondition=PV.Vdc  SampleTime=10*Ts  HasFrameUpgradeWarning=on
  ZOH/3 : ZeroOrderHold  SampleTime=100*Ts
  start MPPT Voltage : Constant  Value=PV.Vdc  SampleTime=Ts
  Vmpp : Outport  VectorParamsAs1DForOutWhenUnconnected=off
  wires:
  OR/1 -> Switch4/2
  Compare To Zero1/1 -> NOR/1, AND1/2
  start MPPT Voltage/1 -> Switch5/3
  Compare To Zero2/1 -> NOR/2, AND1/1
  Pref/1 -> Unit Delay/1, Sum/1
  Switch5/1 -> Add/1, Subtract5/2
  Constant1/1 -> Add/2, Subtract5/1
  Vdc/1 -> Switch5/2, Switch5/1, Sum1/2, Unit Delay1/1
  Unit Delay1/1 -> Sum1/1
  Add/1 -> [Vinc]  "INC"
  NOR/1 -> OR/2
  Subtract5/1 -> [Vdec]  "DEC"
  [Vdec] -> Switch4/3
  Switch4/1 -> ZOH/3/1
  Sum1/1 -> Compare To Zero1/1
  Sum/1 -> Compare To Zero2/1
  AND1/1 -> OR/1
  Unit Delay/1 -> Sum/2
  ZOH/3/1 -> Vmpp/1
  [Vinc] -> Switch4/1

== system remoteMicrogrid/Diesel Substation, BESS, & Microgrid Controller/Microgrid Controller/Resynchronization to Diesel/Frequency and voltage matching/Synch Voltage/Subsystem2 ==
  MicrogridController : Inport
  ControlRoom : Inport  Port=2
  Constant : Constant
  Switch : Switch  Criteria=u2 > Threshold  Threshold=0.5  SaturateOnIntegerOverflow=off  InputSameDT=off
  SynchVoltage : Outport
  wires:
  Switch/1 -> SynchVoltage/1
  Constant/1 -> Switch/3
  MicrogridController/1 -> Switch/1
  ControlRoom/1 -> Switch/2
